simulink model "sampleModel2053"  (R2023a)
settings: Solver=VariableStepAuto  StartTime=0.0  StopTime=10.0  RelTol=1e-3
libraries: hdlsllib x3, simulink x3
settings Model: Creator=user1  LastModifiedBy=user1

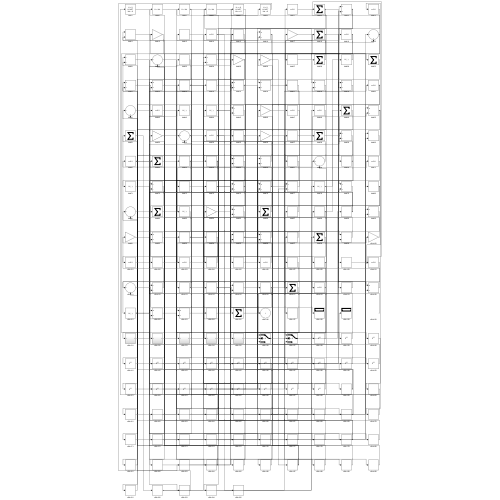
[thumbnail: Simulink's stored preview of the top-level diagram]
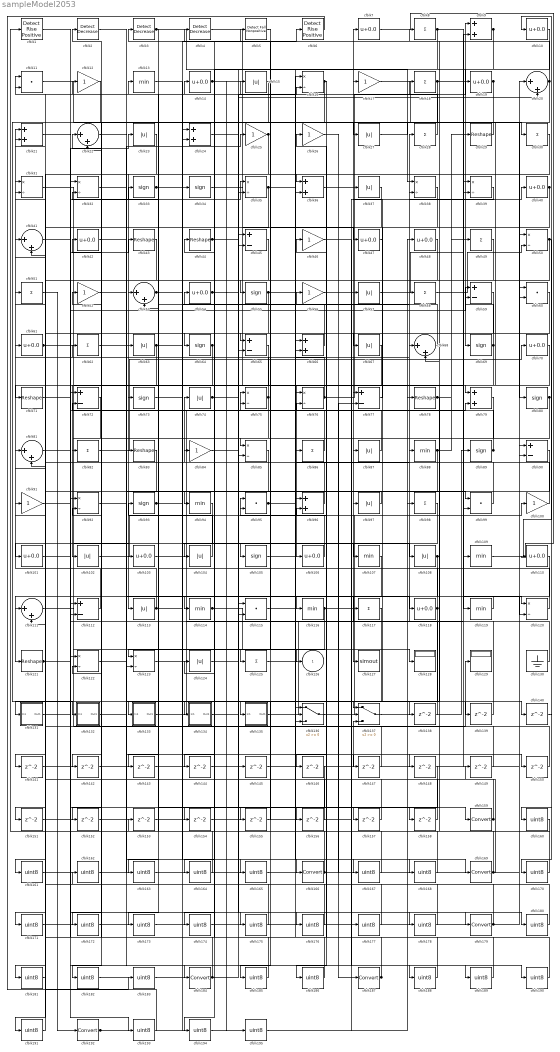
== system sampleModel2053 ==
  cfblk1 : hdlsllib/Logic and Bit Operations/Detect Rise Positive  vinit=0  OutDataTypeStr=boolean
  cfblk{7,10,14,19,40,42,47..48,54,61,70,101,103,106,110,118} (16 alike) : Bias  Bias=0.0  SaturateOnIntegerOverflow=off
  cfblk{12,17,25..26,46,52,56,84,91,100} (10 alike) : Gain
  cfblk{15,23,27,37,57,63,67,74,87,97,102,104,108,113,124} (15 alike) : Abs  SaturateOnIntegerOverflow=off
  cfblk{33..34,55,64,69,73,80,89,93,105} (10 alike) : Signum
  cfblk{13,88,94,107,109,114,116,119} (8 alike) : MinMax
  cfblk{11,60,95,99,115} (5 alike) : DotProduct  OutDataTypeStr=Inherit: Inherit via internal rule
  cfblk{20,22,41,53,68,81,111} (7 alike) : Sum  Inputs=|++
  cfblk{45,59,65,72,77,90,112} (7 alike) : Sum  Inputs=+-
  cfblk{8,18,28,30,49,51,58,62,82,86,98,117,125} (13 alike) : Sum  Inputs=+
  cfblk{16,31..32,35,38..39,50,75..76,85,92,120,122..123} (14 alike) : Product  Inputs=*/  RndMeth=Zero  SaturateOnIntegerOverflow=on
  cfblk{29,43..44,71,78,83,121} (7 alike) : Reshape
  cfblk127 : ToWorkspace  VariableName=simout  SaveFormat=Timeseries  SampleTime=-1
  cfblk128 : Display
  cfblk129 : Display
  cfblk130 : Ground
  cfblk131 : Subsystem
      settings: LibrarySourceBlock=|
      | hdlsllib/Ports &
      | Subsystems/Subsystem
  cfblk132 : Subsystem
      settings: LibrarySourceBlock=|
      | hdlsllib/Ports &
      | Subsystems/Subsystem
  cfblk133 : Subsystem
      settings: LibrarySourceBlock=|
      | hdlsllib/Ports &
      | Subsystems/Subsystem
  cfblk134 : Subsystem
      settings: LibrarySourceBlock=|
      | hdlsllib/Ports &
      | Subsystems/Subsystem
  cfblk135 : Subsystem
      settings: LibrarySourceBlock=|
      | hdlsllib/Ports &
      | Subsystems/Subsystem
  cfblk136 : Switch  SaturateOnIntegerOverflow=off  InputSameDT=off
  cfblk137 : Switch  SaturateOnIntegerOverflow=off  InputSameDT=off
  cfblk{138..158} (21 alike) : Delay  SampleTime=1
  cfblk{159,166,169,179,184,187,192} (7 alike) : DataTypeConversion  SaturateOnIntegerOverflow=off  RndMeth=Floor
  cfblk{160..165,167..168,170..178,180..183,185..186,188..191,193..195} (30 alike) : DataTypeConversion  OutDataTypeStr=uint8  SaturateOnIntegerOverflow=off  RndMeth=Floor
  cfblk2 : simulink/Logic and Bit Operations/Detect Decrease  vinit=0.0  OutDataTypeStr=boolean
      settings: LibrarySourceBlock=|
      | hdlsllib/Logic and Bit
      | Operations/Detect
      | Decrease
  cfblk{9,21,24,36,66,79,96} (7 alike) : Sum
  cfblk3 : simulink/Logic and Bit Operations/Detect Decrease  vinit=0.0  OutDataTypeStr=boolean
      settings: LibrarySourceBlock=|
      | hdlsllib/Logic and Bit
      | Operations/Detect
      | Decrease
  cfblk4 : simulink/Logic and Bit Operations/Detect Decrease  vinit=0.0  OutDataTypeStr=boolean
      settings: LibrarySourceBlock=|
      | hdlsllib/Logic and Bit
      | Operations/Detect
      | Decrease
  cfblk5 : hdlsllib/Logic and Bit Operations/Detect Fall Nonpositive  vinit=0  OutDataTypeStr=boolean
  cfblk6 : hdlsllib/Logic and Bit Operations/Detect Rise Positive  vinit=0  OutDataTypeStr=boolean
  cfblk126 : Outport  VectorParamsAs1DForOutWhenUnconnected=off
  wires:
  cfblk108/1 -> cfblk116/1, cfblk8/1
  cfblk9/1 -> cfblk69/1, cfblk136/3
  cfblk133/1(Out1) -> cfblk75/1
  cfblk92/1 -> cfblk166/1
  cfblk114/1 -> cfblk128/1, cfblk178/1
  cfblk82/1 -> cfblk70/1
  cfblk14/1 -> cfblk106/1, cfblk195/1
  cfblk102/1 -> cfblk95/1
  cfblk25/1 -> cfblk113/1, cfblk134/1(In1)
  cfblk78/1 -> cfblk135/1(In1), cfblk29/1
  cfblk72/1 -> cfblk129/1
  cfblk97/1 -> cfblk94/1
  cfblk125/1 -> cfblk7/1
  cfblk55/1 -> cfblk65/1, cfblk168/1
  cfblk43/1 -> cfblk53/1
  cfblk135/1(Out1) -> cfblk28/1
  cfblk31/1 -> cfblk103/1
  cfblk112/1 -> cfblk21/1
  cfblk70/1 -> cfblk114/1
  cfblk137/1 -> cfblk89/1
  cfblk103/1 -> cfblk50/1
  cfblk80/1 -> cfblk104/1, cfblk152/1
  cfblk12/1 -> cfblk132/1(In1)
  cfblk74/1 -> cfblk20/2, cfblk140/1
  cfblk107/1 -> cfblk121/1
  cfblk136/1 -> cfblk100/1
  cfblk27/1 -> cfblk30/1
  cfblk121/1 -> cfblk75/2, cfblk79/2
  cfblk131/1(Out1) -> cfblk43/1
  cfblk130/1 -> cfblk87/1
  cfblk123/1 -> cfblk39/1
  cfblk89/1 -> cfblk17/1, cfblk22/2
  cfblk119/1 -> cfblk111/1
  cfblk63/1 -> cfblk102/1, cfblk58/1
  cfblk19/1 -> cfblk154/1, cfblk182/1
  cfblk17/1 -> cfblk39/2
  cfblk41/1 -> cfblk23/1
  cfblk53/1 -> cfblk133/1(In1), cfblk150/1
  cfblk105/1 -> cfblk68/1
  cfblk75/1 -> cfblk13/1, cfblk83/1
  cfblk132/1(Out1) -> cfblk25/1
  cfblk122/1 -> cfblk184/1
  cfblk79/1 -> cfblk86/1
  cfblk76/1 -> cfblk18/1, cfblk31/1
  cfblk104/1 -> cfblk53/2
  cfblk116/1 -> cfblk123/1, cfblk40/1
  cfblk120/1 -> cfblk56/1
  cfblk58/1 -> cfblk50/2
  cfblk88/1 -> cfblk96/1, cfblk49/1
  cfblk86/1 -> cfblk14/1
  cfblk84/1 -> cfblk179/1
  cfblk36/1 -> cfblk9/1
  cfblk35/1 -> cfblk71/1, cfblk148/1
  cfblk83/1 -> cfblk111/2
  cfblk64/1 -> cfblk82/1, cfblk151/1
  cfblk99/1 -> cfblk41/2
  cfblk28/1 -> cfblk11/1
  cfblk1/1 -> cfblk159/1
  cfblk4/1 -> cfblk119/1
  cfblk66/1 -> cfblk32/2
  cfblk118/1 -> cfblk93/1, cfblk191/1
  cfblk10/1 -> cfblk64/1
  cfblk3/1 -> cfblk38/1, cfblk73/1
  cfblk87/1 -> cfblk22/1
  cfblk134/1(Out1) -> cfblk97/1
  cfblk47/1 -> cfblk137/1
  cfblk96/1 -> cfblk74/1
  cfblk106/1 -> cfblk5/1
  cfblk61/1 -> cfblk109/1, cfblk35/1, cfblk31/2
  cfblk110/1 -> cfblk127/1
  cfblk5/1 -> cfblk55/1
  cfblk37/1 -> cfblk125/1
  cfblk24/1 -> cfblk169/1
  cfblk109/1 -> cfblk10/1
  cfblk11/1 -> cfblk80/1
  cfblk32/1 -> cfblk99/1
  cfblk56/1 -> cfblk117/1
  cfblk39/1 -> cfblk38/2
  cfblk33/1 -> cfblk155/1, cfblk156/1
  cfblk16/1 -> cfblk35/2, cfblk146/1
  cfblk68/1 -> cfblk4/1
  cfblk100/1 -> cfblk62/1
  cfblk111/1 -> cfblk126/1
  cfblk13/1 -> cfblk105/1
  cfblk101/1 -> cfblk59/1
  cfblk57/1 -> cfblk19/1
  cfblk113/1 -> cfblk72/2, cfblk158/1
  cfblk26/1 -> cfblk187/1
  cfblk69/1 -> cfblk123/2, cfblk59/2
  cfblk62/1 -> cfblk118/1
  cfblk8/1 -> cfblk120/1, cfblk65/2
  cfblk50/1 -> cfblk131/1(In1), cfblk170/1
  cfblk51/1 -> cfblk192/1
  cfblk34/1 -> cfblk47/1
  cfblk18/1 -> cfblk120/2, cfblk85/2
  cfblk7/1 -> cfblk110/1
  cfblk93/1 -> cfblk6/1, cfblk107/1
  cfblk23/1 -> cfblk112/2
  cfblk40/1 -> cfblk67/1, cfblk85/1
  cfblk44/1 -> cfblk16/2, cfblk76/1
  cfblk54/1 -> cfblk108/1, cfblk145/1
  cfblk95/1 -> cfblk88/1, cfblk77/1
  cfblk29/1 -> cfblk27/1
  cfblk20/1 -> cfblk36/1, cfblk3/1, cfblk79/1
  cfblk77/1 -> cfblk37/1
  cfblk94/1 -> cfblk101/1
  cfblk124/1 -> cfblk115/1
  cfblk49/1 -> cfblk115/2
  cfblk2/1 -> cfblk138/1
  cfblk138/1 -> cfblk112/1
  cfblk52/1 -> cfblk139/1
  cfblk139/1 -> cfblk32/1
  cfblk59/1 -> cfblk141/1
  cfblk141/1 -> cfblk99/2
  cfblk67/1 -> cfblk142/1
  cfblk85/1 -> cfblk143/1
  cfblk143/1 -> cfblk9/2
  cfblk65/1 -> cfblk144/1
  cfblk144/1 -> cfblk20/1
  cfblk145/1 -> cfblk137/3
  cfblk42/1 -> cfblk147/1
  cfblk147/1 -> cfblk41/1
  cfblk149/1 -> cfblk96/2
  cfblk150/1 -> cfblk136/2
  cfblk151/1 -> cfblk137/2
  cfblk153/1 -> cfblk136/1
  cfblk154/1 -> cfblk36/2
  cfblk155/1 -> cfblk95/2
  cfblk156/1 -> cfblk21/2
  cfblk115/1 -> cfblk157/1
  cfblk157/1 -> cfblk66/1
  cfblk158/1 -> cfblk12/1
  cfblk159/1 -> cfblk15/1, cfblk72/1
  cfblk140/1 -> cfblk160/1
  cfblk160/1 -> cfblk1/1
  cfblk60/1 -> cfblk161/1
  cfblk161/1 -> cfblk63/1
  cfblk162/1 -> cfblk60/1
  cfblk148/1 -> cfblk163/1
  cfblk163/1 -> cfblk60/2
  cfblk48/1 -> cfblk164/1
  cfblk164/1 -> cfblk33/1
  cfblk73/1 -> cfblk165/1
  cfblk165/1 -> cfblk48/1
  cfblk166/1 -> cfblk153/1, cfblk77/2, cfblk188/1
  cfblk152/1 -> cfblk167/1
  cfblk167/1 -> cfblk92/1
  cfblk168/1 -> cfblk92/2
  cfblk169/1 -> cfblk149/1, cfblk68/2
  cfblk170/1 -> cfblk24/1
  cfblk30/1 -> cfblk171/1
  cfblk171/1 -> cfblk24/2
  cfblk90/1 -> cfblk172/1
  cfblk172/1 -> cfblk66/2
  cfblk15/1 -> cfblk173/1
  cfblk173/1 -> cfblk90/1
  cfblk146/1 -> cfblk174/1
  cfblk174/1 -> cfblk90/2
  cfblk91/1 -> cfblk175/1
  cfblk175/1 -> cfblk42/1
  cfblk71/1 -> cfblk176/1
  cfblk176/1 -> cfblk91/1
  cfblk46/1 -> cfblk177/1
  cfblk177/1 -> cfblk44/1
  cfblk178/1 -> cfblk46/1
  cfblk179/1 -> cfblk162/1, cfblk124/1
  cfblk22/1 -> cfblk180/1
  cfblk180/1 -> cfblk84/1
  cfblk45/1 -> cfblk181/1
  cfblk181/1 -> cfblk61/1
  cfblk182/1 -> cfblk45/1
  cfblk6/1 -> cfblk183/1
  cfblk183/1 -> cfblk45/2
  cfblk184/1 -> cfblk52/1, cfblk2/1
  cfblk117/1 -> cfblk185/1
  cfblk185/1 -> cfblk122/1
  cfblk38/1 -> cfblk186/1
  cfblk186/1 -> cfblk122/2
  cfblk187/1 -> cfblk11/2, cfblk76/2, cfblk16/1
  cfblk188/1 -> cfblk26/1
  cfblk81/1 -> cfblk189/1
  cfblk189/1 -> cfblk54/1
  cfblk142/1 -> cfblk190/1
  cfblk190/1 -> cfblk81/1
  cfblk191/1 -> cfblk81/2
  cfblk192/1 -> cfblk78/1, cfblk34/1
  cfblk21/1 -> cfblk193/1
  cfblk193/1 -> cfblk51/1
  cfblk98/1 -> cfblk194/1
  cfblk194/1 -> cfblk57/1
  cfblk195/1 -> cfblk98/1

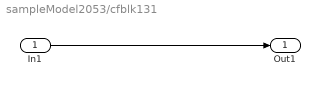
== system sampleModel2053/cfblk131 ==
  In1 : Inport
  Out1 : Outport
  wires:
  In1/1 -> Out1/1

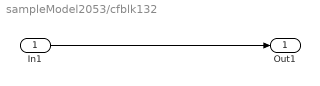
== system sampleModel2053/cfblk132 ==
  In1 : Inport
  Out1 : Outport
  wires:
  In1/1 -> Out1/1

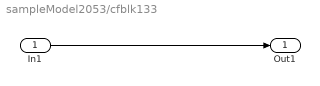
== system sampleModel2053/cfblk133 ==
  In1 : Inport
  Out1 : Outport
  wires:
  In1/1 -> Out1/1

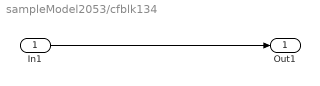
== system sampleModel2053/cfblk134 ==
  In1 : Inport
  Out1 : Outport
  wires:
  In1/1 -> Out1/1

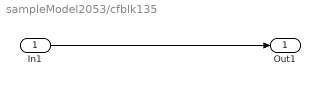
== system sampleModel2053/cfblk135 ==
  In1 : Inport
  Out1 : Outport
  wires:
  In1/1 -> Out1/1
